simulink model "AutopilotModeLogic"  (R2023b)
settings: Solver=FixedStepDiscrete  StartTime=0.0  StopTime=8  FixedStep=Sample_time  RelTol=1e-3
undefined symbols (not defined in the file): Sample_time
Description:
  | Illustrative autopilot mode-management training logic with OFF, ARMED, ENGAGED, and DEGRADED states.
settings Model: DataDictionary=FCS_Data.sldd  Creator=Tyler  LastModifiedBy=Tyler
settings CodeAppCC: MaxIdLength=63

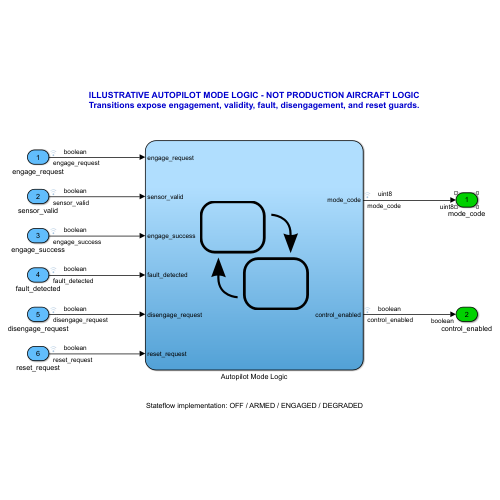
[thumbnail: Simulink's stored preview of the top-level diagram]
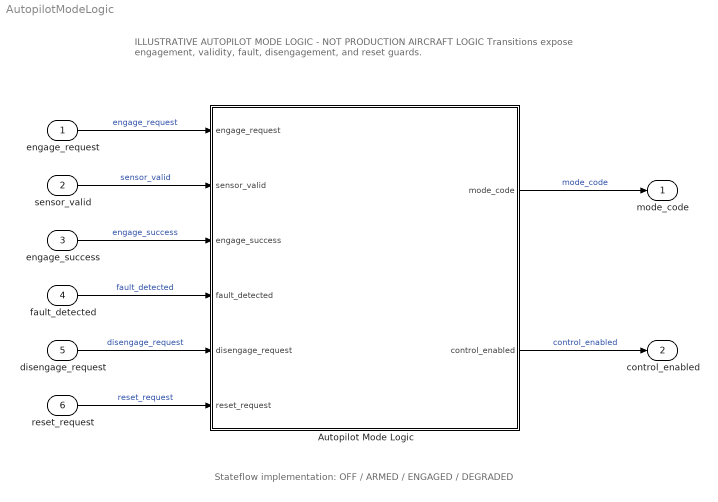
== system AutopilotModeLogic ==
  note: ILLUSTRATIVE AUTOPILOT MODE LOGIC - NOT PRODUCTION AIRCRAFT LOGIC
      | Transitions expose engagement, validity, fault, disengagement, and reset guards.
  note: Stateflow implementation: OFF / ARMED / ENGAGED / DEGRADED
  engage_request : Inport  OutDataTypeStr=boolean  Unit=1  SampleTime=Sample_time
  sensor_valid : Inport  Port=2  OutDataTypeStr=boolean  Unit=1  SampleTime=Sample_time
  engage_success : Inport  Port=3  OutDataTypeStr=boolean  Unit=1  SampleTime=Sample_time
  fault_detected : Inport  Port=4  OutDataTypeStr=boolean  Unit=1  SampleTime=Sample_time
  disengage_request : Inport  Port=5  OutDataTypeStr=boolean  Unit=1  SampleTime=Sample_time
  reset_request : Inport  Port=6  OutDataTypeStr=boolean  Unit=1  SampleTime=Sample_time
  Autopilot Mode Logic : Stateflow chart  TreatAsAtomicUnit=on
  mode_code : Outport  OutDataTypeStr=uint8  Unit=1
  control_enabled : Outport  Port=2  OutDataTypeStr=boolean  Unit=1
  wires:
  engage_request/1 -> Autopilot Mode Logic/1(engage_request)  "engage_request"
  sensor_valid/1 -> Autopilot Mode Logic/2(sensor_valid)  "sensor_valid"
  engage_success/1 -> Autopilot Mode Logic/3(engage_success)  "engage_success"
  fault_detected/1 -> Autopilot Mode Logic/4(fault_detected)  "fault_detected"
  disengage_request/1 -> Autopilot Mode Logic/5(disengage_request)  "disengage_request"
  reset_request/1 -> Autopilot Mode Logic/6(reset_request)  "reset_request"
  Autopilot Mode Logic/1(mode_code) -> mode_code/1  "mode_code"
  Autopilot Mode Logic/2(control_enabled) -> control_enabled/1  "control_enabled"

== stateflow chart AutopilotModeLogic/Autopilot Mode Logic ==
  settings: description=Illustrative training mode state machine. mode_code mapping: OFF=0, ARMED=1, ENGAGED=2, DEGRADED=3.
  state OFF
    entry:
    mode_code = uint8(0);
    control_enabled = false;
  state ARMED
    entry:
    mode_code = uint8(1);
    control_enabled = false;
  state DEGRADED
    entry:
    mode_code = uint8(3);
    control_enabled = false;
  state ENGAGED
    entry:
    mode_code = uint8(2);
    control_enabled = true;
  (junction 24) -> (junction 26)
  (default) -> OFF
  (junction 21) -> (junction 24)
  (junction 26) -> OFF
  ARMED -> OFF [order 3] : [disengage_request]
  OFF -> ARMED : [engage_request && sensor_valid]
  DEGRADED -> OFF : [reset_request || disengage_request]
  ARMED -> (junction 28) [order 2]
  ARMED -> ENGAGED [order 1] : [engage_success && sensor_valid]
  (junction 28) -> (junction 30) : [fault_detected || ~sensor_valid]
  (junction 30) -> DEGRADED
  ENGAGED -> DEGRADED [order 1] : [fault_detected || ~sensor_valid]
  ENGAGED -> (junction 21) [order 2] : [disengage_request]
  data: engage_request input boolean; sensor_valid input boolean; engage_success input boolean; fault_detected input boolean; disengage_request input boolean; reset_request input boolean; mode_code output uint8; control_enabled output boolean
